simulink model "Logic_control"  (R2023a)
settings: Solver=ode23t  StartTime=0.0  StopTime=3  MaxStep=0.01  RelTol=1e-4
undefined symbols (not defined in the file): Linear_part
settings Model: Creator=ПК  LastModifiedBy=ПК

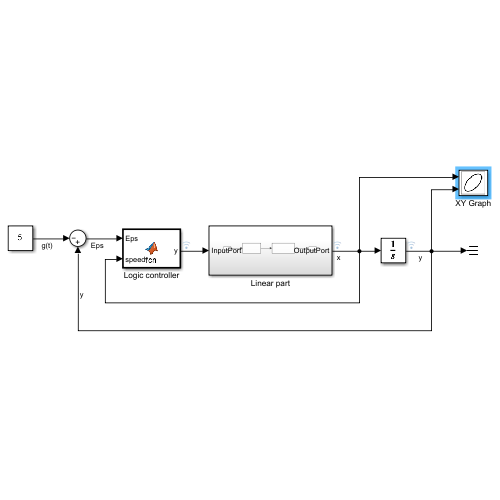
[thumbnail: Simulink's stored preview of the top-level diagram]
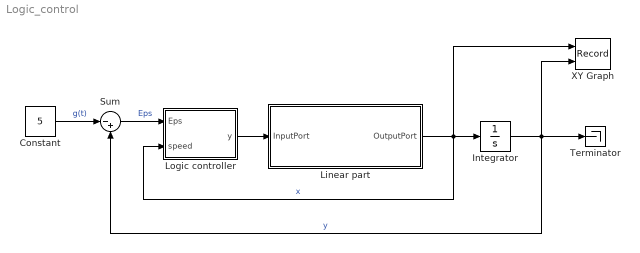
== system Logic_control ==
  Constant : Constant  Value=5
  Integrator : Integrator
  Linear part : Subsystem
  Logic controller : MATLAB Function  TreatAsAtomicUnit=on
  Sum : Sum  Inputs=|-+
  Terminator : Terminator
  XY Graph : Record  FileSettingsInternal="{\"entries\":[{\"content\":{\"excelSettings\":{\"content\":{},\"type\":\"Streamout.ExcelSettings\"}},\"type\":\"Streamout.FileSettingStorage\",\"uuid\":\"cb6f7f12-1d2c-4e6b-ac47-1a0cbdb01e3e\"}],\"packageUris\":[\"http://schema.mathworks.com/mf0/streamout_blocks/R2020a\"],\"version\":\"1.0\"}"  Layout=[1 1]  SignalsInternal="{\"entries\":[{\"content\":{\"signals\":[{\"content\":{\"blockPath\":[\"Logic_control/XY Graph\"],\"dimensions\":[1],\"domain\":\"Logic_control/XY Graph\",\"lineColor\":\"#a2142f\",\"plots\":[1],\"port\":1,\"sid\":[\"\"],\"signalID\":2662,\"signalName\":\"x\"},\"type\":\"RecordBlkView.Signal\",\"uuid\":\"01f015c5-33fb-4f62-8e8e-825978a93b81\"},{\"content\":{\"blockPath\":[\"Logic_control/XY Graph\"],\"dimensions\":[1],\"domain\":\"Logic_control/XY Graph\",\"lineColor\":\"#139fff\",\"plots\":[1],\"port\":2,\"sid\":[\"\"],\"signalID\":2666,\"signalName\":\"y\"},\"type\":\"RecordBlkView.Signal\",\"uuid\":\"12dfc569-2d08-4992-84ee-57eca047f93b\"}]},\"type\":\"RecordBlkView.InputSignals\",\"uuid\":\"f70e7319-39e3-43b1-941f-68caa420815e\"}],\"packageUris\":[\"http://schema.mathworks.com/mf0/streamout_blocks/R2020a\"],\"version\":\"1.0\"}"  VisualizationBindings="{\"xyplotplugin\":{\"info\":[{\"series\":[{\"bindingParametersList\":[{\"parameter\":\"X-Axis\",\"signalID\":2662,\"signalName\":\"x\"},{\"parameter\":\"Y-Axis\",\"signalID\":2666,\"signalName\":\"y\"}],\"seriesID\":42852}],\"subplotID\":1}]}}"  CompatibilityTag=XY
  wires:
  Constant/1 -> Sum/1  "g(t)"
  Linear part/1(OutputPort) -> XY Graph/1, Logic controller/2(speed), Integrator/1  "x"
  Sum/1 -> Logic controller/1(Eps)  "Eps"
  Integrator/1 -> XY Graph/2, Terminator/1, Sum/2  "y"
  Logic controller/1(y) -> Linear part/1(InputPort)

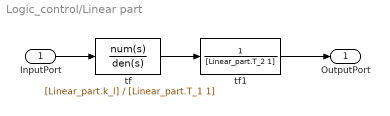
== system Logic_control/Linear part ==
  InputPort : Inport
  tf : TransferFcn  Numerator=[Linear_part.k_l]  Denominator=[Linear_part.T_1 1]
  tf1 : TransferFcn  Denominator=[Linear_part.T_2 1]
  OutputPort : Outport
  wires:
  InputPort/1 -> tf/1
  tf/1 -> tf1/1
  tf1/1 -> OutputPort/1

== matlab function Logic_control/Logic controller ==
  data: Eps input; y output; speed input
function y = fcn(Eps, speed)

a_1 = 0.5;
a_2 = 2;

if ( Eps < -a_1 ) && (speed < -a_2)
    y = 1;
elseif ( Eps < -a_1 ) && (speed < a_2)
    y = 1;
elseif ( Eps > a_1 ) && (speed < a_2)
    y = -1;
elseif ( Eps > a_1 ) && (speed > a_2)
    y = -1;
else
    y = 0;
end
